simulink model "untitled1"  (R2021a)
settings: Solver=VariableStepAuto  StartTime=0.0  StopTime=10.0  RelTol=1e-3
settings Model: Creator=HP  LastModifiedBy=ASUS

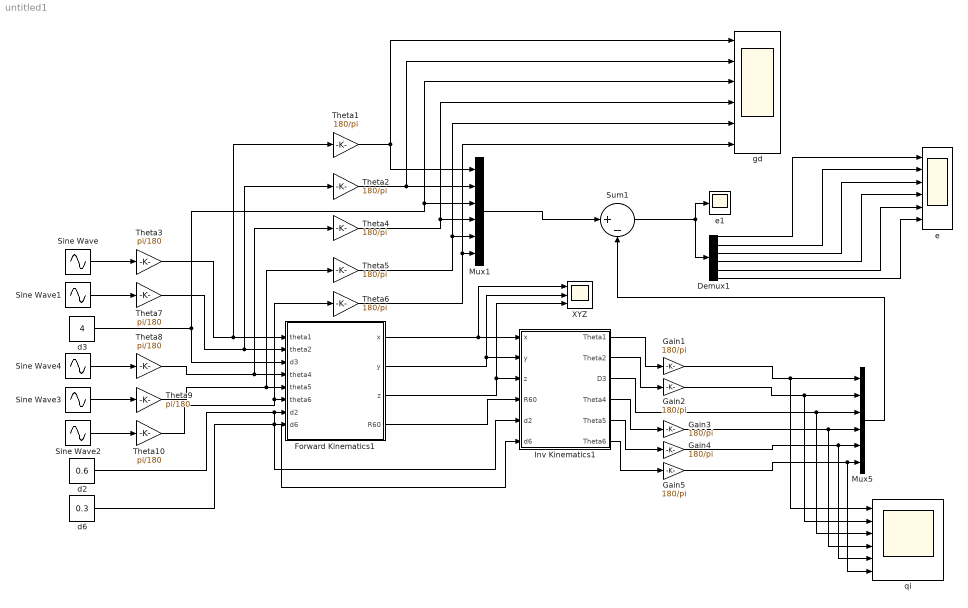
== system untitled1 ==
  Demux1 : Demux  Outputs=6
  Forward Kinematics1 : Subsystem
  Gain{1..5} (5 alike) : Gain  Gain=180/pi
  Inv Kinematics1 : Subsystem
  Mux1 : Mux  Inputs=6
  Mux5 : Mux  Inputs=6
  Sine Wave{,1..4} (5 alike) : Sin  SampleTime=0
  Sum1 : Sum  Inputs=|+-
  Theta{1..2,4..6} (5 alike) : Gain  Gain=180/pi
  Theta{3,7..10} (5 alike) : Gain  Gain=pi/180
  XYZ : Scope  NumInputPorts=3
  d2 : Constant  Value=0.6
  d3 : Constant  Value=4
  d6 : Constant  Value=0.3
  e : Scope  NumInputPorts=6
  e1 : Scope
  gd : Scope  NumInputPorts=6
  qi : Scope  NumInputPorts=6
  wires:
  Sine Wave/1 -> Theta3/1
  Sine Wave1/1 -> Theta7/1
  Sine Wave4/1 -> Theta8/1
  Sine Wave3/1 -> Theta9/1
  Sine Wave2/1 -> Theta10/1
  d2/1 -> Inv Kinematics1/5(d2), Forward Kinematics1/7(d2)
  d6/1 -> Inv Kinematics1/6(d6), Forward Kinematics1/8(d6)
  Forward Kinematics1/1(x) -> XYZ/1, Inv Kinematics1/1(x)
  Forward Kinematics1/2(y) -> Inv Kinematics1/2(y), XYZ/2
  Forward Kinematics1/3(z) -> XYZ/3, Inv Kinematics1/3(z)
  Forward Kinematics1/4(R60) -> Inv Kinematics1/4(R60)
  Inv Kinematics1/1(Theta1) -> Gain1/1
  Inv Kinematics1/2(Theta2) -> Gain2/1
  Inv Kinematics1/4(Theta4) -> Gain3/1
  Inv Kinematics1/5(Theta5) -> Gain4/1
  Inv Kinematics1/6(Theta6) -> Gain5/1
  Gain1/1 -> Mux5/1, qi/1
  Gain2/1 -> Mux5/2, qi/2
  Gain3/1 -> Mux5/4, qi/4
  Gain4/1 -> Mux5/5, qi/5
  Gain5/1 -> qi/6, Mux5/6
  Inv Kinematics1/3(D3) -> Mux5/3, qi/3
  Theta2/1 -> Mux1/2, gd/2
  Theta6/1 -> gd/6, Mux1/6
  Theta5/1 -> Mux1/5, gd/5
  Theta4/1 -> Mux1/4, gd/4
  Mux1/1 -> Sum1/1
  Demux1/6 -> e/6
  Demux1/5 -> e/5
  Sum1/1 -> e1/1, Demux1/1
  Demux1/4 -> e/4
  Demux1/2 -> e/2
  Demux1/1 -> e/1
  Demux1/3 -> e/3
  Theta1/1 -> gd/1, Mux1/1
  d3/1 -> Forward Kinematics1/3(d3), Mux1/3, gd/3
  Mux5/1 -> Sum1/2
  Theta3/1 -> Forward Kinematics1/1(theta1), Theta1/1
  Theta7/1 -> Forward Kinematics1/2(theta2), Theta2/1
  Theta8/1 -> Forward Kinematics1/4(theta4), Theta4/1
  Theta9/1 -> Theta5/1, Forward Kinematics1/5(theta5)
  Theta10/1 -> Theta6/1, Forward Kinematics1/6(theta6)

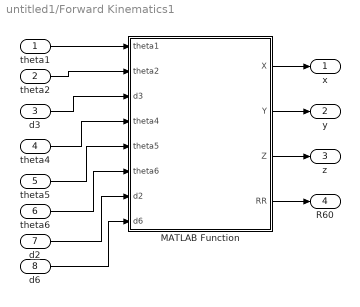
== system untitled1/Forward Kinematics1 ==
  theta1 : Inport
  theta2 : Inport  Port=2
  d3 : Inport  Port=3
  theta4 : Inport  Port=4
  theta5 : Inport  Port=5
  theta6 : Inport  Port=6
  d2 : Inport  Port=7
  d6 : Inport  Port=8
  MATLAB Function : MATLAB Function  TreatAsAtomicUnit=on
  x : Outport
  y : Outport  Port=2
  z : Outport  Port=3
  R60 : Outport  Port=4
  wires:
  MATLAB Function/1(X) -> x/1
  MATLAB Function/2(Y) -> y/1
  MATLAB Function/3(Z) -> z/1
  theta1/1 -> MATLAB Function/1(theta1)
  theta2/1 -> MATLAB Function/2(theta2)
  d3/1 -> MATLAB Function/3(d3)
  theta4/1 -> MATLAB Function/4(theta4)
  theta5/1 -> MATLAB Function/5(theta5)
  theta6/1 -> MATLAB Function/6(theta6)
  d2/1 -> MATLAB Function/7(d2)
  MATLAB Function/4(RR) -> R60/1
  d6/1 -> MATLAB Function/8(d6)

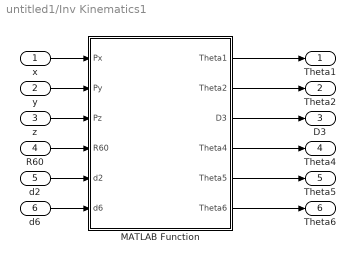
== system untitled1/Inv Kinematics1 ==
  x : Inport
  y : Inport  Port=2
  z : Inport  Port=3
  R60 : Inport  Port=4
  d2 : Inport  Port=5
  d6 : Inport  Port=6
  MATLAB Function : MATLAB Function  TreatAsAtomicUnit=on
  Theta1 : Outport
  Theta2 : Outport  Port=2
  D3 : Outport  Port=3
  Theta4 : Outport  Port=4
  Theta5 : Outport  Port=5
  Theta6 : Outport  Port=6
  wires:
  y/1 -> MATLAB Function/2(Py)
  x/1 -> MATLAB Function/1(Px)
  MATLAB Function/1(Theta1) -> Theta1/1
  MATLAB Function/2(Theta2) -> Theta2/1
  z/1 -> MATLAB Function/3(Pz)
  MATLAB Function/3(D3) -> D3/1
  R60/1 -> MATLAB Function/4(R60)
  d2/1 -> MATLAB Function/5(d2)
  d6/1 -> MATLAB Function/6(d6)
  MATLAB Function/4(Theta4) -> Theta4/1
  MATLAB Function/5(Theta5) -> Theta5/1
  MATLAB Function/6(Theta6) -> Theta6/1

== matlab function untitled1/Forward Kinematics1/MATLAB Function ==
  data: theta1 input; theta2 input; d3 input; theta4 input; X output; Y output; Z output; theta5 input; theta6 input; d2 input; RR output; d6 input


function [X,Y,Z,RR]  = fcn(theta1,theta2,d3,theta4,theta5,theta6,d2,d6)

[X,Y,Z,RR] = STANFORD_Forward_Kinematics(theta1,theta2,d3,theta4,theta5,theta6,d2,d6);

== matlab function untitled1/Inv Kinematics1/MATLAB Function ==
  data: Px input; Py input; Theta1 output; Theta2 output; Pz input; D3 output; R60 input; d2 input; d6 input; Theta4 output; Theta5 output; Theta6 output


function [Theta1,Theta2,D3,Theta4,Theta5,Theta6]=fcn(Px,Py,Pz,R60,d2,d6)

[Theta1,Theta2,D3,Theta4,Theta5,Theta6]=STANFORD_InverseKinematics(Px,Py,Pz,R60,d2,d6)
